simulink model "EKF_trial_on_PX4_2023a"  (R2023b)
settings: Solver=VariableStepAuto  StartTime=0.0  StopTime=10.0  RelTol=1e-3
values from neighbouring files (symbols this model uses):
  Kv = [-0.0025558316857  0.000132590019729  0.000149679484256; 0.000145839006277  -0.00203404256706  -9.11330285567e-05; 0.000381907915659  -0.000223412194351  -0.00502920519016]    [K_pole_inv.mat]    (also in quadcopterMain.m = K(end))
  Kx = [0.0400138549738 -0.00118949210727 -0.00296492634583 -0.00108295834628 0.0357572143705 0.00174392641634 -0.00117611344216 0.000709574560023 0.0795788253978 0.157190780188 -0.00011499619581 -0.000286465619495 ... (18 elements, 3x6)]    [K_pole_inv.mat]    (also in quadcopterMain.m = K(1:6))
  P0 = diag([P0_ph_meas,P0_th_meas,P0_ps_meas,P0_bias_wp,P0_bias_wq,P0_bias_wr])    [EKF.m]
  param = [Ixx;Iyy;Izz;l;k;b;m]    [main_matteo.m]    (also in quadcopterMain.m)
  Q = diag([q_phi,q_theta,q_psi, q_bias_w_b,q_bias_w_b,q_bias_w_b])    [EKF.m]
  R = diag([r_th_meas,r_th_meas,r_ps_meas])    [EKF.m]
  Rbody_frd = [cos(angleZ) -sin(angleZ)   0 ... (first row only)    [EKF.m]
  Rbody_ned = Rbody_frd*Rfrd_ned    [EKF.m]
  Ts_EKF_integr = 0.01    [EKF.m]
  Ts_EKF_meas = 0.01    [EKF.m]
  Ts_slk = 0.01    [main_matteo.m]    (also in quadcopterMain.m)
  x0EKF = [ph0;th0;ps0;bias_wp0;bias_wq0;bias_wr0]    [EKF.m]
undefined symbols (not defined in the file or in its folder): DiscIntNeverNeededParam, mf
settings Model: Creator=teoma  LastModifiedBy=teoma

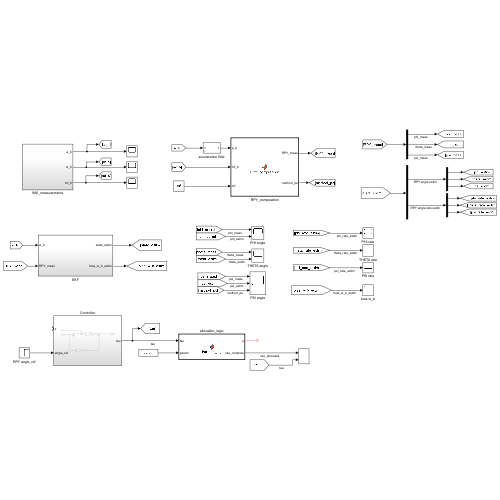
[thumbnail: Simulink's stored preview of the top-level diagram]
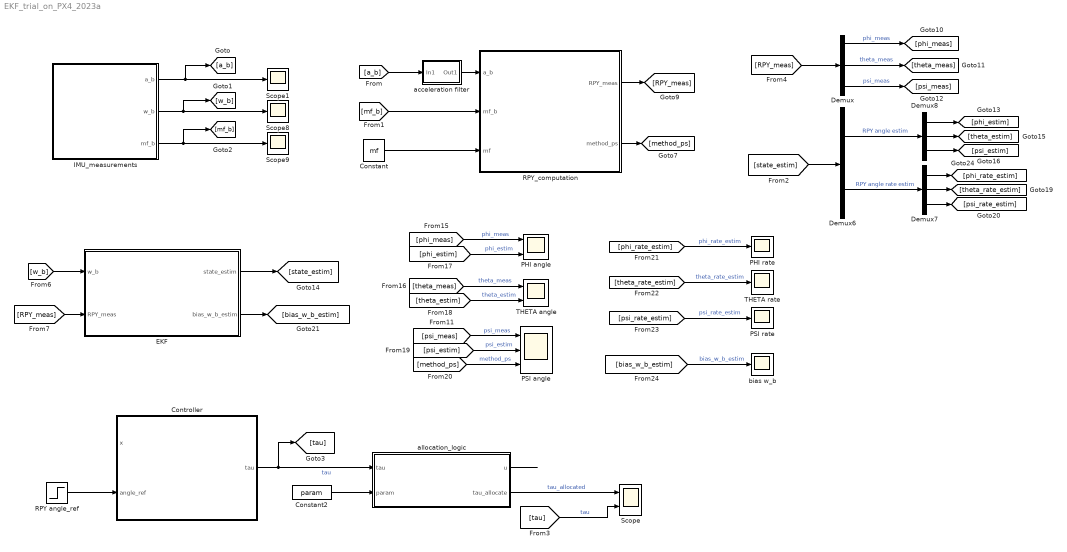
== system EKF_trial_on_PX4_2023a ==
  Constant : Constant  Value=mf
  Constant2 : Constant  Value=param
  Controller : Subsystem
  Demux : Demux  Outputs=3
  Demux6 : Demux  Outputs=2
  Demux7 : Demux  Outputs=3
  Demux8 : Demux  Outputs=3
  EKF : Subsystem
  IMU_measurements : Subsystem
  PHI angle : Scope  NumInputPorts=2
  PHI rate : Scope
  PSI angle : Scope  NumInputPorts=3
  PSI rate : Scope
  RPY angle_ref : Step  Time=20  After=[0.52;0.52;0.52]  SampleTime=0
  RPY_computation : MATLAB Function  TreatAsAtomicUnit=on
  Scope : Scope  NumInputPorts=2
  Scope1 : Scope
  Scope8 : Scope
  Scope9 : Scope
  THETA angle : Scope  NumInputPorts=2
  THETA rate : Scope
  acceleration filter : Subsystem  mask{p=5}
      mask prompts: p "pole"
  allocation_logic : MATLAB Function  TreatAsAtomicUnit=on
  bias w_b : Scope
  wires:
  [mf_b] -> RPY_computation/2(mf_b)
  RPY_computation/2(method_ps) -> [method_ps]
  [a_b] -> acceleration filter/1(In1)
  RPY_computation/1(RPY_meas) -> [RPY_meas]
  Constant/1 -> RPY_computation/3(mf)
  acceleration filter/1(Out1) -> RPY_computation/1(a_b)
  [RPY_meas] -> EKF/2(RPY_meas)
  EKF/2(bias_w_b_estim) -> [bias_w_b_estim]
  EKF/1(state_estim) -> [state_estim]
  [w_b] -> EKF/1(w_b)
  IMU_measurements/2(w_b) -> Scope8/1, [w_b]
  IMU_measurements/1(a_b) -> [a_b], Scope1/1
  IMU_measurements/3(mf_b) -> [mf_b], Scope9/1
  Demux6/1 -> Demux8/1  "RPY angle estim"
  Demux8/2 -> [theta_estim]
  Demux8/1 -> [phi_estim]
  [RPY_meas] -> Demux/1
  Demux/1 -> [phi_meas]  "phi_meas"
  Demux7/2 -> [theta_rate_estim]
  Demux/2 -> [theta_meas]  "theta_meas"
  Demux7/1 -> [phi_rate_estim]
  [state_estim] -> Demux6/1
  Demux8/3 -> [psi_estim]
  Demux/3 -> [psi_meas]  "psi_meas"
  Demux6/2 -> Demux7/1  "RPY angle rate estim"
  Demux7/3 -> [psi_rate_estim]
  [phi_estim] -> PHI angle/2  "phi_estim"
  [phi_meas] -> PHI angle/1  "phi_meas"
  [method_ps] -> PSI angle/3  "method_ps"
  [psi_estim] -> PSI angle/2  "psi_estim"
  [psi_meas] -> PSI angle/1  "psi_meas"
  [theta_meas] -> THETA angle/1  "theta_meas"
  [theta_estim] -> THETA angle/2  "theta_estim"
  [bias_w_b_estim] -> bias w_b/1  "bias_w_b_estim"
  [phi_rate_estim] -> PHI rate/1  "phi_rate_estim"
  [theta_rate_estim] -> THETA rate/1  "theta_rate_estim"
  [psi_rate_estim] -> PSI rate/1  "psi_rate_estim"
  allocation_logic/2(tau_allocate) -> Scope/1  "tau_allocated"
  Constant2/1 -> allocation_logic/2(param)
  Controller/1(tau) -> allocation_logic/1(tau), [tau]  "tau"
  allocation_logic/1(u) -> ?
  RPY angle_ref/1 -> Controller/2(angle_ref)
  [tau] -> Scope/2  "tau"

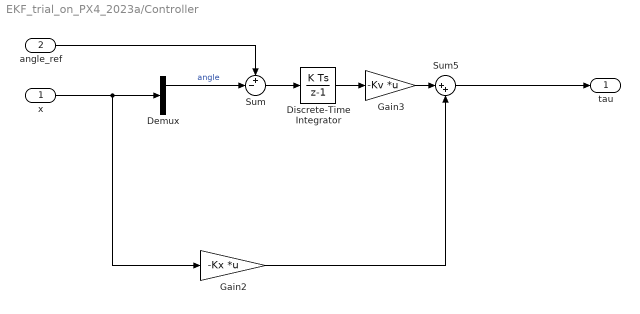
== system EKF_trial_on_PX4_2023a/Controller ==
  x : Inport
  angle_ref : Inport  Port=2
  Demux : Demux  Outputs=2
  Discrete-Time Integrator : DiscreteIntegrator  SampleTime=Ts_slk  ICPrevOutput=DiscIntNeverNeededParam  ICPrevScaledInput=DiscIntNeverNeededParam
  Gain2 : Gain  Gain=-Kx  Multiplication=Matrix(K*u)
  Gain3 : Gain  Gain=-Kv  Multiplication=Matrix(K*u)
  Sum : Sum  Inputs=+-|
  Sum5 : Sum  Inputs=|++
  tau : Outport
  wires:
  x/1 -> Gain2/1, Demux/1
  Sum5/1 -> tau/1
  angle_ref/1 -> Sum/1
  Discrete-Time Integrator/1 -> Gain3/1
  Sum/1 -> Discrete-Time Integrator/1
  Gain3/1 -> Sum5/1
  Demux/1 -> Sum/2  "angle"
  Gain2/1 -> Sum5/2

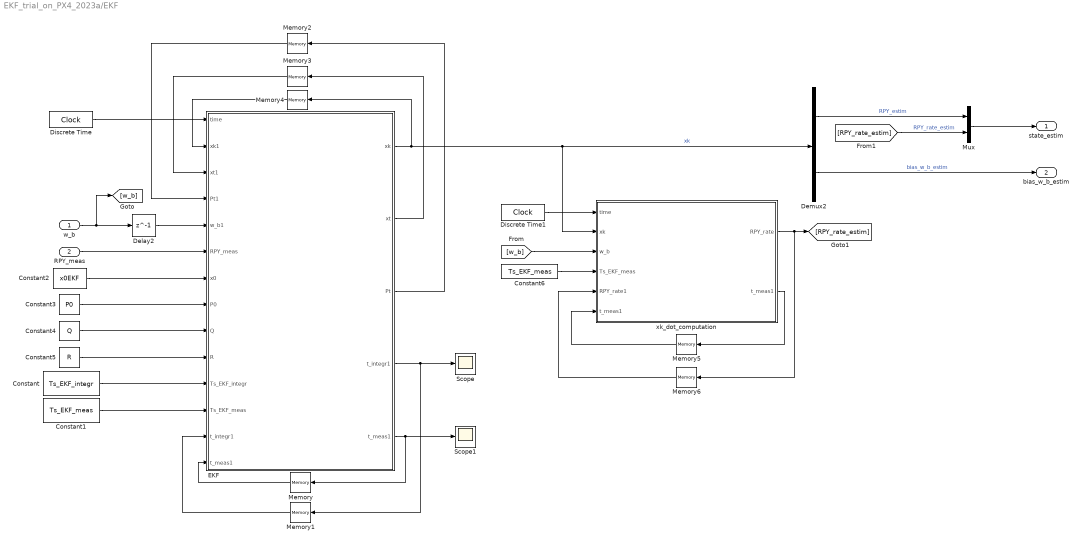
== system EKF_trial_on_PX4_2023a/EKF ==
  w_b : Inport
  RPY_meas : Inport  Port=2
  Constant : Constant  Value=Ts_EKF_integr
  Constant1 : Constant  Value=Ts_EKF_meas
  Constant2 : Constant  Value=x0EKF
  Constant3 : Constant  Value=P0
  Constant4 : Constant  Value=Q
  Constant5 : Constant  Value=R
  Constant6 : Constant  Value=Ts_EKF_meas
  Delay2 : Delay  DelayLength=1  SampleTime=Ts_EKF_integr
  Demux2 : Demux  Outputs=2
  Discrete Time : DigitalClock  SampleTime=Ts_slk
  Discrete Time1 : DigitalClock  SampleTime=Ts_slk
  EKF : MATLAB Function  TreatAsAtomicUnit=on
  Memory{,1..6} (7 alike) : Memory
  Mux : Mux  Inputs=2
  Scope : Scope
  Scope1 : Scope
  xk_dot_computation : MATLAB Function  TreatAsAtomicUnit=on
  state_estim : Outport
  bias_w_b_estim : Outport  Port=2
  wires:
  w_b/1 -> Delay2/1, [w_b]
  Constant4/1 -> EKF/9(Q)
  Constant2/1 -> EKF/7(x0)
  Constant5/1 -> EKF/10(R)
  Memory/1 -> EKF/14("t_meas1 ")
  EKF/2(xt) -> Memory3/1
  Memory2/1 -> EKF/4(Pt1)
  EKF/3(Pt) -> Memory2/1
  RPY_meas/1 -> EKF/6(RPY_meas)
  Discrete Time/1 -> EKF/1(time)
  Memory3/1 -> EKF/3(xt1)
  Memory1/1 -> EKF/13("t_integr1 ")
  Constant3/1 -> EKF/8(P0)
  EKF/5(t_meas1) -> Scope1/1, Memory/1
  EKF/4(t_integr1) -> Scope/1, Memory1/1
  Delay2/1 -> EKF/5(w_b1)
  Constant/1 -> EKF/11(Ts_EKF_integr)
  Constant1/1 -> EKF/12(Ts_EKF_meas)
  Memory4/1 -> EKF/2(xk1)
  xk_dot_computation/2(t_meas1) -> Memory5/1
  Memory5/1 -> xk_dot_computation/6("t_meas1 ")
  Memory6/1 -> xk_dot_computation/5(RPY_rate1)
  xk_dot_computation/1(RPY_rate) -> [RPY_rate_estim], Memory6/1
  [w_b] -> xk_dot_computation/3(w_b)
  Discrete Time1/1 -> xk_dot_computation/1(time)
  Demux2/2 -> bias_w_b_estim/1  "bias_w_b_estim"
  Demux2/1 -> Mux/1  "RPY_estim"
  EKF/1(xk) -> xk_dot_computation/2(xk), Demux2/1, Memory4/1  "xk"
  [RPY_rate_estim] -> Mux/2  "RPY_rate_estim"
  Mux/1 -> state_estim/1
  Constant6/1 -> xk_dot_computation/4(Ts_EKF_meas)

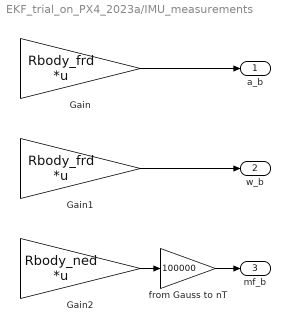
== system EKF_trial_on_PX4_2023a/IMU_measurements ==
  Gain : Gain  Gain=Rbody_frd  Multiplication=Matrix(K*u) (u vector)
  Gain1 : Gain  Gain=Rbody_frd  Multiplication=Matrix(K*u) (u vector)
  Gain2 : Gain  Gain=Rbody_ned  Multiplication=Matrix(K*u) (u vector)
  from Gauss to nT : Gain  Gain=100000
  a_b : Outport
  w_b : Outport  Port=2
  mf_b : Outport  Port=3
  wires:
  Gain/1 -> a_b/1
  Gain1/1 -> w_b/1
  from Gauss to nT/1 -> mf_b/1
  Gain2/1 -> from Gauss to nT/1
  ? -> Gain2/1

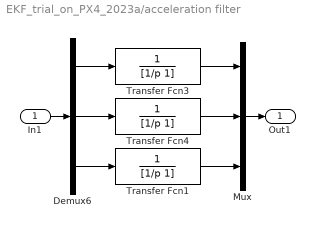
== system EKF_trial_on_PX4_2023a/acceleration filter ==
  In1 : Inport
  Demux6 : Demux  Outputs=3
  Mux : Mux  Inputs=3
  Transfer Fcn1 : TransferFcn  Denominator=[1/p 1]
  Transfer Fcn3 : TransferFcn  Denominator=[1/p 1]
  Transfer Fcn4 : TransferFcn  Denominator=[1/p 1]
  Out1 : Outport
  wires:
  Transfer Fcn4/1 -> Mux/2
  Demux6/3 -> Transfer Fcn1/1
  Mux/1 -> Out1/1
  Transfer Fcn1/1 -> Mux/3
  Transfer Fcn3/1 -> Mux/1
  In1/1 -> Demux6/1
  Demux6/1 -> Transfer Fcn3/1
  Demux6/2 -> Transfer Fcn4/1

== matlab function EKF_trial_on_PX4_2023a/RPY_computation ==
  data: a_b input; mf_b input; RPY_meas output; mf input; method_ps output
function [RPY_meas,method_ps]   = RPY_computation(a_b,mf_b,mf)
% description:
% - a_b             = measured linear acceleration in body-frame
% - w_b             = measured angular velocity in body-frame
% - mf_b            = measured magnetic field in body-frame
% - mf              = measured magnetic field in body-inertia
% - a_b_disturbe    = linear velocity measurement-noise
% - w_b_disturbe    = angular velocity measurement-noise
% - mf_b_disturbe   = magnetic field measurement-noise

% -------------------------------------------------------------------------------------------
% observation: the following computation works only if the angles
% phi,theta,psy are withing angles (-pi/2,+pi/2) (this is an open set, pi/2 is excluded)
% -------------------------------------------------------------------------------------------

a_b = -1*a_b;       % need to adjust the sign to use atan2() function correctly
mf_u = mf(3,1);     % magnetic field in up direction (z-dir in inertia frame)

% phi computation
ph_meas = atan2(a_b(2), a_b(3));
sph = sin(ph_meas);
cph = cos(ph_meas);

% theta computation
th_meas = atan2(-a_b(1), (a_b(2)*sph + a_b(3)*cph));
sth = sin(th_meas);
cth = cos(th_meas);

% psi computation
if abs(sin(th_meas)) > 0.1  % sin(th) != 0 
    method_ps = 1;
    ps_meas_numerator   = (sth*cph*mf_b(2) - sth*sph*mf_b(3))/(-sth);       % don't modify
    ps_meas_denominator = (-sph*mf_b(2) - cph*mf_b(3) + cth*mf_u)/(-sth);   % don't modify
    ps_meas = atan2(ps_meas_numerator, ps_meas_denominator);
else                        % sin(th) == 0
    method_ps = 2;
    ps_meas_numerator   = (mf_b(2) - cth*sph*mf_u)*(-cth);
    ps_meas_denominator = cph*mf_b(1);
    ps_meas = atan2(ps_meas_numerator, ps_meas_denominator);
end
RPY_meas = [ph_meas;th_meas;ps_meas];

== matlab function EKF_trial_on_PX4_2023a/EKF/EKF ==
  data: time input; xk1 input; xt1 input; Pt1 input; w_b1 input; RPY_meas input; x0 input; P0 input; Q input; R input; Ts_EKF_integr input; Ts_EKF_meas input; xk output; t_integr1 input; t_meas1 input; xt output; Pt output; t_integr1 output; t_meas1 output
function [xk,xt,Pt,t_integr1,t_meas1] = EKF(time,xk1,xt1,Pt1,w_b1,RPY_meas,x0,P0,Q,R,Ts_EKF_integr,Ts_EKF_meas,t_integr1,t_meas1)

if time == 0
    xk = x0;
    xt = x0;
    Pt = P0;
    t_integr1 = 0;
    t_meas1 = 0;
elseif time - t_integr1 >= Ts_EKF_integr
    wp          =       w_b1(1,1);        % p-dir of angular velocity w
    wq          =       w_b1(2,1);        % q-dir of angular velocity w
    wr          =       w_b1(3,1);        % r-dir of angular velocity w

    phi         =       xt1(1,1);         %  roll angle (rad)
    theta       =       xt1(2,1);         %  pitch angle (rad)
    psi         =       xt1(3,1);         %  yaw angle (rad)  
    bias_wp     =       xt1(4,1);         % bias of p-dir of angular velocity w
    bias_wq     =       xt1(5,1);         % bias of q-dir of angular velocity w
    bias_wr     =       xt1(6,1);         % bias of r-dir of angular velocity w

    cph         =       cos(phi);
    cth         =       cos(theta);
    cps         =       cos(psi);
    sph         =       sin(phi);
    sth         =       sin(theta);
    sps         =       sin(psi);
    tth         =       sth/cth;

    % integration step
    t_integr1 = time;
    Mf = [1,    sph*tth,    cph*tth,    0,  0,  0;
          0,    cph,        -sph,       0,  0,  0;
          0,    sph/cth,    cph/cth,    0,  0,  0;
          0,    0,          0,          1,  0,  0;
          0,    0,          0,          0,  1,  0;
          0,    0,          0,          0,  0,  1;];
    Z1 = [wp-bias_wp; wq-bias_wq; wr-bias_wr; bias_wp; bias_wq; bias_wr;];
    f = Mf*Z1;
    xt = xt1 + Ts_EKF_integr*f;

    A1 = [cph*tth*(wq-bias_wq)-sph*tth*(wr-bias_wr),(sph*(wq-bias_wq)+cph*(wr-bias_wr))/cth^2,  0,  -1, -sph*tth,   -cph*tth;];
    A2 = [-sph*(wq-bias_wq)-cph*(wr-bias_wr),   0,  0,  0,  -cph,   sph;];
    A3 = [cph*(wq-bias_wq)/cth-sph*(wr-bias_wr)/cth, (sth/cth^2)*(sph*(wq-bias_wq)+cph*(wr-bias_wr)),   0,  0,  -sph/cth,   -cph/cth;];
    A4 = [0,    0,  0,  1,  0,  0;];
    A5 = [0,    0,  0,  0,  1,  0;];
    A6 = [0,    0,  0,  0,  0,  1;];
    At1 = [A1; A2; A3; A4; A5; A6;];
    Pt = Pt1 + Ts_EKF_integr*(At1*Pt1 + Pt1*At1' + Q);

    % measurement step
    if time - t_meas1 >= Ts_EKF_meas
        t_meas1 = time;
        Ck = [eye(3),zeros(3,3)];
        Lk = Pt*Ck'/(Ck*Pt*Ck' + R);
        xk = xt + Lk*(RPY_meas - Ck*xt);
        Pk = (eye(6) - Lk*Ck)*Pt;

        xt = xk;    % becomes the new xt1
        Pt = Pk;    % becomes the new Pt1
    else
        xk = xk1;    % xk1
    end
else
    xk = xt1;
    xt = xt1;
    Pt = Pt1;
end
end

== matlab function EKF_trial_on_PX4_2023a/EKF/xk_dot_computation ==
  data: time input; xk input; w_b input; Ts_EKF_meas input; RPY_rate1 input; RPY_rate output; t_meas1 input; t_meas1 output
function [RPY_rate,t_meas1] = xk_dot_computation(time,xk,w_b,Ts_EKF_meas,RPY_rate1,t_meas1)
RPY_rate = zeros(3,1);
if time == 0
    t_meas1 = 0;
end
if time - t_meas1 >= Ts_EKF_meas || time == 0
    wp          =       w_b(1,1);        % p-dir of angular velocity w
    wq          =       w_b(2,1);        % q-dir of angular velocity w
    wr          =       w_b(3,1);        % r-dir of angular velocity w

    phi         =       xk(1,1);         %  roll angle (rad)
    theta       =       xk(2,1);         %  pitch angle (rad)
    psi         =       xk(3,1);         %  yaw angle (rad)  
    bias_wp     =       xk(4,1)*0;         % bias of p-dir of angular velocity w
    bias_wq     =       xk(5,1)*0;         % bias of q-dir of angular velocity w
    bias_wr     =       xk(6,1)*0;         % bias of r-dir of angular velocity w

    cph         =       cos(phi);
    cth         =       cos(theta);
    cps         =       cos(psi);
    sph         =       sin(phi);
    sth         =       sin(theta);
    sps         =       sin(psi);
    tth         =       sth/cth;

    % integration step
    t_meas1 = time;
    W_eta = [1,    sph*tth,    cph*tth;
             0,    cph,        -sph;
             0,    sph/cth,    cph/cth;];
    w_b_corrected = [wp-bias_wp; wq-bias_wq; wr-bias_wr;];
    RPY_rate = W_eta*w_b_corrected;
else
    RPY_rate = RPY_rate1;
end
end

== matlab function EKF_trial_on_PX4_2023a/allocation_logic ==
  data: tau input; u output; param input; tau_allocate output
function [u, tau_allocate] = allocation_logic(tau,param)
% Allocation Logic Block: computes the corresponding control command
% u = [u1,u2,u3,u4] given the torque command tau = [tau_phi, tau_theta, tau_phi]

% control command limits
u_min = 0;
u_max = 1000;

l = param(4,1);
k = param(5,1);
b = param(6,1);

% [tau_ph; tau_th; tau_ps]' = Mtau_u * [u1;u2;u3;u4]
Mtau_u = [0      0       l*k     -l*k;
          -l*k   l*k     0       0;
          -b     -b      b       b;];
Minv = Mtau_u'*inv(Mtau_u*Mtau_u');
up = Minv*tau;
un = zeros(4,1);
if min(up(:)) < u_min 
    un = ones(4,1)*(u_min - min(up(:)));
end
u = up+un;
for i = 1:1:4
    if u(i,1) > u_max
        u(i,1) = u_max;
    end
end
 tau_allocate = Mtau_u*u;
